simulink library "NG_Genset_lib"  (Simulink 8.1)
settings: Solver=ode45  StartTime=0.0  StopTime=10.0  RelTol=1e-3
undefined symbols (not defined in the file): fdesignblkfcn, gcbh, ph, Ts
libraries: simulink x24, rtio_opalrt_common x21, simulink_extras x6, powerlib x4, rteventslib x4, GEJenbacherJ620_lib x2
(part 3 of 3)

== system NG_Genset_lib/NG_3_5_MVA_Generator/NG Genset 3.5MVA1/3.5MVA Generator with  Primary Controllers1/NG Engine Speed & Voltage Control fast/Excitation1 ==
  note: link disabled
  note: link disabled
  vref : Inport
  v : Inport  Port=2
  vstab : Inport  Port=3
  Damping kf.s / (tf.s +1) : Subsystem
  Exciter  1 / (te.s + ke) : Subsystem
  Lead Lag Compensator tc.s+1 / tb.s+1 : Subsystem  AncestorBlock=|  mask(Discrete Lead-Lag Controller){T1=tgr(2), T2=tgr(1), V_Init=exc(1)*v0(2)/reg(1), Ts=Ts}
      | powerlib_extras/Discrete 
      | Control Blocks/Discrete
      | Lead-Lag
      mask prompts: T1 "Time constant T1 (s):"; T2 "Time constant T2 (s):"; V_Init "Initial input and output:"; Ts "Sample time (s):"
      mask help:
      | This block implements a discrete lead-lag controller:
      |
      |          1+T1s
      | H(s)= ------
      |          1+T2s
      |
      | States are initialized according to initial input anf output value so that simulation starts in steady state.
      mask init: same as NG_Genset_lib/NG Genset 3.5MVA/3.5MVA Generator with  Primary Controllers1/NG Engine Speed & Voltage Control fast/Excitation1/Lead Lag Compensator tc.s+1 / tb.s+1
      mask Display: disp('1+T1s\n---\n1+T2s')
  Low Pass Filter 1 / (tr.s +1) (with IC) : Subsystem  AncestorBlock=|  mask(Discrete 1st-Order Filter){FilterType=Lowpass, Tc=tr, Ts=Ts, Initialize=on, Vac_Init=[0 0 60], Vdc_Init=v0(1), PlotResponse=off, param1=[1 500 0.1]}
      | powerlib_extras/Discrete 
      | Control Blocks/Discrete
      | 1st-Order
      | Discrete Filter
      mask prompts: FilterType "Filter Type:"; Tc "Time constant (s):"; Ts "Sample time:"; Initialize "Initialize filter states"; Vac_Init "AC initial input: [ Mag  Phase(degrees)  Freq(Hz) ]"; Vdc_Init "DC Initial input:"; PlotResponse "Plot filter response"; param1 "Frequency range(Hz) : [Start  End  Inc.]"
      mask init: same as NG_Genset_lib/NG Genset 3.5MVA/3.5MVA Generator with  Primary Controllers1/NG Engine Speed & Voltage Control fast/Excitation1/Low Pass Filter 1 / (tr.s +1) (with IC)
      mask TypeOptions FilterType: Lowpass | Highpass
      mask Callback Initialize: p4=get_param(gcb,'Initialize');if strcmp(p4,'on');visible={'on','on','on','on','on','on','on',get_param(gcb,'PlotResponse')};else;visible={'on','on','on','on','off','off','on',get_param(gcb,'PlotResponse')};end;set_param(gcb,'MaskVisibilities',visible)
      mask Callback PlotResponse: p7=get_param(gcb,'PlotResponse');if strcmp(p7,'on');visible={'on','on','on','on',get_param(gcb,'Initialize'),get_param(gcb,'Initialize'),'on','on'};else;visible={'on','on','on','on',get_param(gcb,'Initialize'),get_param(gcb,'Initialize'),'on','off'};end;set_param(gcb,'MaskVisibilities',visible)
      mask Display: plot(X,Y);
  Main Regulator ka / (ta.s +1) : Subsystem
  Sum : Sum  Inputs=++-+-  SaturateOnIntegerOverflow=on  InputSameDT=on  OutDataTypeStr=Inherit: Same as first input
  Unit Delay1 : UnitDelay  SampleTime=Ts
  Unit Delay2 : UnitDelay  InitialCondition=v0(2)  SampleTime=Ts
  Vf0 / ka : Constant  Value=v0(2)/reg(1)
  proportional saturation : Subsystem
  Vf1 : Outport  InitialOutput=0
  wires:
  Unit Delay2/1 -> Vf1/1
  Unit Delay1/1 -> Sum/5
  proportional saturation/1(Ef) -> Exciter  1 / (te.s + ke)/1(In)
  Lead Lag Compensator tc.s+1 / tb.s+1/1(Out1) -> Main Regulator ka / (ta.s +1)/1(In)
  Sum/1 -> Lead Lag Compensator tc.s+1 / tb.s+1/1(In1)
  v/1 -> Low Pass Filter 1 / (tr.s +1) (with IC)/1(In)
  vref/1 -> Sum/1
  vstab/1 -> Sum/4
  Low Pass Filter 1 / (tr.s +1) (with IC)/1(Out) -> proportional saturation/2(Vtf), Sum/3
  Vf0 / ka/1 -> Sum/2
  Main Regulator ka / (ta.s +1)/1(Out) -> proportional saturation/1(Efd)
  Damping kf.s / (tf.s +1)/1(Out) -> Unit Delay1/1
  Exciter  1 / (te.s + ke)/1(Out) -> Unit Delay2/1, Damping kf.s / (tf.s +1)/1(In)

== system NG_Genset_lib/NG Genset 3.5MVA/3.5MVA Generator with  Primary Controllers1/NG Engine Speed & Voltage Control fast/Excitation1/Damping kf.s / (tf.s +1)/1st-Order Discrete Filter ==
  In : Inport
  Discrete State-Space : DiscreteStateSpace  A=Ad  B=Bd  C=Cd  D=Dd  X0=x0d  SampleTime=Ts
  Out : Outport  InitialOutput=0
  wires:
  Discrete State-Space/1 -> Out/1
  In/1 -> Discrete State-Space/1

== system NG_Genset_lib/NG Genset 3.5MVA/3.5MVA Generator with  Primary Controllers1/NG Engine Speed & Voltage Control fast/Excitation1/Exciter  1 / (te.s + ke)/1st order Lowpass ==
  In : Inport
  Discrete State-Space : DiscreteStateSpace  A=Ad  B=Bd  C=Cd  D=Dd  X0=x0d  SampleTime=Ts
  Out : Outport  InitialOutput=0
  wires:
  Discrete State-Space/1 -> Out/1
  In/1 -> Discrete State-Space/1

== system NG_Genset_lib/NG Genset 3.5MVA/3.5MVA Generator with  Primary Controllers1/NG Engine Speed & Voltage Control fast/Excitation1/Main Regulator ka / (ta.s +1)/1st order Lowpass ==
  In : Inport
  Discrete State-Space : DiscreteStateSpace  A=Ad  B=Bd  C=Cd  D=Dd  X0=x0d  SampleTime=Ts
  Out : Outport  InitialOutput=0
  wires:
  Discrete State-Space/1 -> Out/1
  In/1 -> Discrete State-Space/1

== system NG_Genset_lib/NG_3_5_MVA_Generator/NG Genset 3.5MVA1/3.5MVA Generator with  Primary Controllers1/NG Engine Speed & Voltage Control fast/Excitation1/Damping kf.s / (tf.s +1) ==
  note: link disabled
  In : Inport
  1st-Order Discrete Filter : Subsystem  AncestorBlock=|  mask(Discrete 1st-Order Filter){FilterType=Highpass, Tc=damp(2), Ts=Ts, Initialize=on, Vac_Init=[0 0 60], Vdc_Init=damp(1)*v0(2)/damp(2), PlotResponse=off, param1=[1 500 0.1]}
      | powerlib_extras/Discrete 
      | Control Blocks/Discrete
      | 1st-Order
      | Discrete Filter
      mask prompts: FilterType "Filter Type:"; Tc "Time constant (s):"; Ts "Sample time:"; Initialize "Initialize filter states"; Vac_Init "AC initial input: [ Mag  Phase(degrees)  Freq(Hz) ]"; Vdc_Init "DC Initial input:"; PlotResponse "Plot filter response"; param1 "Frequency range(Hz) : [Start  End  Inc.]"
      mask init: same as NG_Genset_lib/NG Genset 3.5MVA/3.5MVA Generator with  Primary Controllers1/NG Engine Speed & Voltage Control fast/Excitation1/Low Pass Filter 1 / (tr.s +1) (with IC)
      mask TypeOptions FilterType: Lowpass | Highpass
      mask Callback Initialize: p4=get_param(gcb,'Initialize');if strcmp(p4,'on');visible={'on','on','on','on','on','on','on',get_param(gcb,'PlotResponse')};else;visible={'on','on','on','on','off','off','on',get_param(gcb,'PlotResponse')};end;set_param(gcb,'MaskVisibilities',visible)
      mask Callback PlotResponse: p7=get_param(gcb,'PlotResponse');if strcmp(p7,'on');visible={'on','on','on','on',get_param(gcb,'Initialize'),get_param(gcb,'Initialize'),'on','on'};else;visible={'on','on','on','on',get_param(gcb,'Initialize'),get_param(gcb,'Initialize'),'on','off'};end;set_param(gcb,'MaskVisibilities',visible)
      mask Display: plot(X,Y);
  Gain : Gain  Gain=damp(1)/damp(2)  SaturateOnIntegerOverflow=on  OutDataTypeStr=Inherit: Same as input  ParamDataTypeStr=Inherit: Same as input
  Out : Outport
  wires:
  1st-Order Discrete Filter/1(Out) -> Out/1
  Gain/1 -> 1st-Order Discrete Filter/1(In)
  In/1 -> Gain/1

== system NG_Genset_lib/NG_3_5_MVA_Generator/NG Genset 3.5MVA1/3.5MVA Generator with  Primary Controllers1/NG Engine Speed & Voltage Control fast/Excitation1/Exciter  1 / (te.s + ke) ==
  note: link disabled
  In : Inport
  1st order Lowpass : Subsystem  AncestorBlock=|  mask(Discrete 1st-Order Filter){FilterType=Lowpass, Tc=exc(2)/exc(1), Ts=Ts, Initialize=on, Vac_Init=[0.0 0 60], Vdc_Init=v0(2), PlotResponse=off, param1=[1 500 0.1]}
      | powerlib_extras/Discrete 
      | Control Blocks/Discrete
      | 1st-Order
      | Discrete Filter
      mask prompts: FilterType "Filter Type:"; Tc "Time constant (s):"; Ts "Sample time:"; Initialize "Initialize filter states"; Vac_Init "AC initial input: [ Mag  Phase(degrees)  Freq(Hz) ]"; Vdc_Init "DC Initial input:"; PlotResponse "Plot filter response"; param1 "Frequency range(Hz) : [Start  End  Inc.]"
      mask init: same as NG_Genset_lib/NG Genset 3.5MVA/3.5MVA Generator with  Primary Controllers1/NG Engine Speed & Voltage Control fast/Excitation1/Low Pass Filter 1 / (tr.s +1) (with IC)
      mask TypeOptions FilterType: Lowpass | Highpass
      mask Callback Initialize: p4=get_param(gcb,'Initialize');if strcmp(p4,'on');visible={'on','on','on','on','on','on','on',get_param(gcb,'PlotResponse')};else;visible={'on','on','on','on','off','off','on',get_param(gcb,'PlotResponse')};end;set_param(gcb,'MaskVisibilities',visible)
      mask Callback PlotResponse: p7=get_param(gcb,'PlotResponse');if strcmp(p7,'on');visible={'on','on','on','on',get_param(gcb,'Initialize'),get_param(gcb,'Initialize'),'on','on'};else;visible={'on','on','on','on',get_param(gcb,'Initialize'),get_param(gcb,'Initialize'),'on','off'};end;set_param(gcb,'MaskVisibilities',visible)
      mask Display: plot(X,Y);
  Gain : Gain  Gain=1/exc(1)  SaturateOnIntegerOverflow=on  OutDataTypeStr=Inherit: Same as input  ParamDataTypeStr=Inherit: Same as input
  Out : Outport
  wires:
  Gain/1 -> 1st order Lowpass/1(In)
  In/1 -> Gain/1
  1st order Lowpass/1(Out) -> Out/1

== system NG_Genset_lib/NG_3_5_MVA_Generator/NG Genset 3.5MVA1/3.5MVA Generator with  Primary Controllers1/NG Engine Speed & Voltage Control fast/Excitation1/Lead Lag Compensator tc.s+1 / tb.s+1 ==
  In1 : Inport
  Discrete State-Space : DiscreteStateSpace  A=Ad  B=Bd  C=Cd  D=Dd  X0=x0d  SampleTime=Ts
  Out1 : Outport
  wires:
  In1/1 -> Discrete State-Space/1
  Discrete State-Space/1 -> Out1/1

== system NG_Genset_lib/NG_3_5_MVA_Generator/NG Genset 3.5MVA1/3.5MVA Generator with  Primary Controllers1/NG Engine Speed & Voltage Control fast/Excitation1/Low Pass Filter 1 / (tr.s +1) (with IC) ==
  In : Inport
  Discrete State-Space : DiscreteStateSpace  A=Ad  B=Bd  C=Cd  D=Dd  X0=x0d  SampleTime=Ts
  Out : Outport  InitialOutput=0
  wires:
  In/1 -> Discrete State-Space/1
  Discrete State-Space/1 -> Out/1

== system NG_Genset_lib/NG_3_5_MVA_Generator/NG Genset 3.5MVA1/3.5MVA Generator with  Primary Controllers1/NG Engine Speed & Voltage Control fast/Excitation1/Main Regulator ka / (ta.s +1) ==
  note: link disabled
  In : Inport
  1st order Lowpass : Subsystem  AncestorBlock=|  mask(Discrete 1st-Order Filter){FilterType=Lowpass, Tc=reg(2), Ts=Ts, Initialize=on, Vac_Init=[0.0 0 60], Vdc_Init=exc(1)*v0(2), PlotResponse=off, param1=[1 500 0.1]}
      | generator_lib/Generator_09222015/GenSet_4MVA_09212015/4MVA Generator with 
      | Primary Controllers1/Diesel Engine
      | Speed & Voltage
      | Control
      | fast/Excitation/Main Regulator
      | ka // (ta.s +1)/1st order
      | Lowpass
      mask prompts: FilterType "Filter Type:"; Tc "Time constant (s):"; Ts "Sample time:"; Initialize "Initialize filter states"; Vac_Init "AC initial input: [ Mag  Phase(degrees)  Freq(Hz) ]"; Vdc_Init "DC Initial input:"; PlotResponse "Plot filter response"; param1 "Frequency range(Hz) : [Start  End  Inc.]"
      mask init: same as NG_Genset_lib/NG Genset 3.5MVA/3.5MVA Generator with  Primary Controllers1/NG Engine Speed & Voltage Control fast/Excitation1/Low Pass Filter 1 / (tr.s +1) (with IC)
      mask TypeOptions FilterType: Lowpass | Highpass
      mask Callback Initialize: p4=get_param(gcb,'Initialize');if strcmp(p4,'on');visible={'on','on','on','on','on','on','on',get_param(gcb,'PlotResponse')};else;visible={'on','on','on','on','off','off','on',get_param(gcb,'PlotResponse')};end;set_param(gcb,'MaskVisibilities',visible)
      mask Callback PlotResponse: p7=get_param(gcb,'PlotResponse');if strcmp(p7,'on');visible={'on','on','on','on',get_param(gcb,'Initialize'),get_param(gcb,'Initialize'),'on','on'};else;visible={'on','on','on','on',get_param(gcb,'Initialize'),get_param(gcb,'Initialize'),'on','off'};end;set_param(gcb,'MaskVisibilities',visible)
      mask Display: plot(X,Y);
  Gain : Gain  Gain=reg(1)  SaturateOnIntegerOverflow=on  OutDataTypeStr=Inherit: Same as input  ParamDataTypeStr=Inherit: Same as input
  Out : Outport
  wires:
  1st order Lowpass/1(Out) -> Out/1
  In/1 -> Gain/1
  Gain/1 -> 1st order Lowpass/1(In)

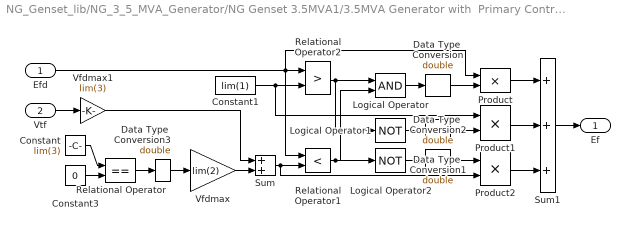
== system NG_Genset_lib/NG_3_5_MVA_Generator/NG Genset 3.5MVA1/3.5MVA Generator with  Primary Controllers1/NG Engine Speed & Voltage Control fast/Excitation1/proportional saturation ==
  Efd : Inport
  Vtf : Inport  Port=2
  Constant : Constant  Value=lim(3)
  Constant1 : Constant  Value=lim(1)
  Constant3 : Constant  Value=0
  Data Type  Conversion{,1..3} (4 alike) : DataTypeConversion  OutDataTypeStr=double  SaturateOnIntegerOverflow=on  RndMeth=Zero
  Logical Operator : Logic
  Logical Operator1 : Logic  Operator=NOT  Inputs=1
  Logical Operator2 : Logic  Operator=NOT  Inputs=1
  Product : Product  SaturateOnIntegerOverflow=on  InputSameDT=on  OutDataTypeStr=Inherit: Same as first input
  Product1 : Product  SaturateOnIntegerOverflow=on  InputSameDT=on  OutDataTypeStr=Inherit: Same as first input
  Product2 : Product  SaturateOnIntegerOverflow=on  InputSameDT=on  OutDataTypeStr=Inherit: Same as first input
  Relational Operator : RelationalOperator  Operator===  InputSameDT=on
  Relational Operator1 : RelationalOperator  Operator=<  InputSameDT=on
  Relational Operator2 : RelationalOperator  Operator=>  InputSameDT=on
  Sum : Sum  SaturateOnIntegerOverflow=on  InputSameDT=on  OutDataTypeStr=Inherit: Same as first input
  Sum1 : Sum  Inputs=+++  SaturateOnIntegerOverflow=on  InputSameDT=on  OutDataTypeStr=Inherit: Same as first input
  Vfdmax : Gain  Gain=lim(2)  SaturateOnIntegerOverflow=on  OutDataTypeStr=Inherit: Same as input  ParamDataTypeStr=Inherit: Same as input
  Vfdmax1 : Gain  Gain=lim(3)  SaturateOnIntegerOverflow=on  OutDataTypeStr=Inherit: Same as input  ParamDataTypeStr=Inherit: Same as input
  Ef : Outport  InitialOutput=0
  wires:
  Data Type  Conversion3/1 -> Vfdmax/1
  Relational Operator/1 -> Data Type  Conversion3/1
  Data Type  Conversion2/1 -> Product2/1
  Logical Operator2/1 -> Data Type  Conversion2/1
  Data Type  Conversion1/1 -> Product1/2
  Logical Operator1/1 -> Data Type  Conversion1/1
  Data Type  Conversion/1 -> Product/2
  Logical Operator/1 -> Data Type  Conversion/1
  Product1/1 -> Sum1/2
  Product2/1 -> Sum1/3
  Product/1 -> Sum1/1
  Sum1/1 -> Ef/1
  Efd/1 -> Product/1, Relational Operator1/1, Relational Operator2/1
  Constant1/1 -> Product1/1, Relational Operator2/2
  Relational Operator1/1 -> Logical Operator/2, Logical Operator2/1
  Relational Operator2/1 -> Logical Operator/1, Logical Operator1/1
  Sum/1 -> Relational Operator1/2, Product2/2
  Vfdmax1/1 -> Sum/1
  Vfdmax/1 -> Sum/2
  Constant3/1 -> Relational Operator/2
  Constant/1 -> Relational Operator/1
  Vtf/1 -> Vfdmax1/1

== system NG_Genset_lib/NG_3_5_MVA_Generator/NG Genset 3.5MVA1/3.5MVA Generator with  Primary Controllers1/NG Engine Speed & Voltage Control fast/Excitation1/Damping kf.s / (tf.s +1)/1st-Order Discrete Filter ==
  In : Inport
  Discrete State-Space : DiscreteStateSpace  A=Ad  B=Bd  C=Cd  D=Dd  X0=x0d  SampleTime=Ts
  Out : Outport  InitialOutput=0
  wires:
  In/1 -> Discrete State-Space/1
  Discrete State-Space/1 -> Out/1

== system NG_Genset_lib/NG_3_5_MVA_Generator/NG Genset 3.5MVA1/3.5MVA Generator with  Primary Controllers1/NG Engine Speed & Voltage Control fast/Excitation1/Exciter  1 / (te.s + ke)/1st order Lowpass ==
  In : Inport
  Discrete State-Space : DiscreteStateSpace  A=Ad  B=Bd  C=Cd  D=Dd  X0=x0d  SampleTime=Ts
  Out : Outport  InitialOutput=0
  wires:
  In/1 -> Discrete State-Space/1
  Discrete State-Space/1 -> Out/1

== system NG_Genset_lib/NG_3_5_MVA_Generator/NG Genset 3.5MVA1/3.5MVA Generator with  Primary Controllers1/NG Engine Speed & Voltage Control fast/Excitation1/Main Regulator ka / (ta.s +1)/1st order Lowpass ==
  In : Inport
  Discrete State-Space : DiscreteStateSpace  A=Ad  B=Bd  C=Cd  D=Dd  X0=x0d  SampleTime=Ts
  Out : Outport  InitialOutput=0
  wires:
  In/1 -> Discrete State-Space/1
  Discrete State-Space/1 -> Out/1
